simulink model "Verification_Tank1_Primitives"  (R2012b)
settings: Solver=FixedStepDiscrete  StartTime=0.0  StopTime=10.0  FixedStep=0.1  RelTol=1e-3
libraries: sldvlib x11
settings Model: Creator=Kerianne  LastModifiedBy=Kerianne
settings DataIOCC: SaveFormat=Structure
settings OptimizationCC: InlineParams=on

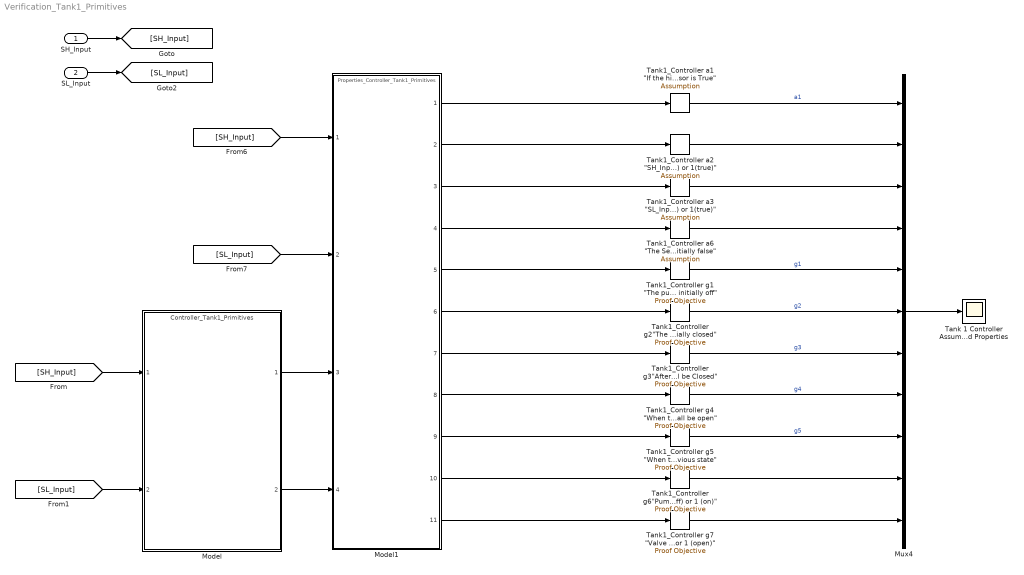
== system Verification_Tank1_Primitives ==
  SH_Input : Inport  OutDataTypeStr=double  SampleTime=0.1
  SL_Input : Inport  Port=2  OutDataTypeStr=double
  Model : ModelReference  ModelNameDialog=Controller_Tank1_Primitives  SimulationMode=Normal  ModelReferenceVersion=1.34  CopyOfModelName=Controller_Tank1_Primitives  DefaultDataLogging=on
  Model1 : ModelReference  ModelNameDialog=Properties_Controller_Tank1_Primitives  SimulationMode=Normal  ModelReferenceVersion=1.40  CopyOfModelName=Properties_Controller_Tank1_Primitives  DefaultDataLogging=on
  Mux4 : Mux  Inputs=11
  Tank 1 Controller Assumptions and Properties : Scope
      settings: ShowLegends=on  YMin=-1  YMax=2
  "Tank1_Controller a1 \"If the high sensor is true, then the low sensor is True\"" : sldvlib/Objectives and Constraints/Assumption  enabled=on  customAVTBlockType=Assumption  intervals=true  initial=off  dispValues=on  outEnabled=on
      settings: AttributesFormatString=%<intervals>
  "Tank1_Controller a2 \"SH_Input is 0 (false) or 1(true)\"" : sldvlib/Objectives and Constraints/Assumption  enabled=on  customAVTBlockType=Assumption  intervals=true  initial=off  dispValues=on  outEnabled=on
      settings: AttributesFormatString=%<intervals>
  "Tank1_Controller a3 \"SL_Input is 0 (false) or 1(true)\"" : sldvlib/Objectives and Constraints/Assumption  enabled=on  customAVTBlockType=Assumption  intervals=true  initial=off  dispValues=on  outEnabled=on
      settings: AttributesFormatString=%<intervals>
  "Tank1_Controller a6 \"The Sensors are initially false\"" : sldvlib/Objectives and Constraints/Assumption  enabled=on  customAVTBlockType=Assumption  intervals=true  initial=off  dispValues=on  outEnabled=on
      settings: AttributesFormatString=%<intervals>
  "Tank1_Controller g1 \"The pump is initially off\"" : sldvlib/Objectives and Constraints/Proof Objective  enabled=on  customAVTBlockType=Proof Objective  intervals=true  dispValues=on  outEnabled=on  enableStopSim=off
      settings: AttributesFormatString=%<intervals>
  "Tank1_Controller g2\"The valve is initially closed\"" : sldvlib/Objectives and Constraints/Proof Objective  enabled=on  customAVTBlockType=Proof Objective  intervals=true  dispValues=on  outEnabled=on  enableStopSim=off
      settings: AttributesFormatString=%<intervals>
  "Tank1_Controller g3\"After the initial time step, When SL_Input is False, the Pump shall be on and Valve shall be Closed\" " : sldvlib/Objectives and Constraints/Proof Objective  enabled=on  customAVTBlockType=Proof Objective  intervals=true  dispValues=on  outEnabled=on  enableStopSim=off
      settings: AttributesFormatString=%<intervals>
  "Tank1_Controller g4 \"When the SH_Input is true, the Pump shall be off and Valve shall be open\"" : sldvlib/Objectives and Constraints/Proof Objective  Description="\"The pump is initially off\""  enabled=on  customAVTBlockType=Proof Objective  intervals=true  dispValues=on  outEnabled=on  enableStopSim=off
      settings: AttributesFormatString=%<intervals>
  "Tank1_Controller g5 \"When the SL_Input is True and the SH_Input is False, the Pump and Valve shall stay in their previous state\"" : sldvlib/Objectives and Constraints/Proof Objective  Tag=g4  enabled=on  customAVTBlockType=Proof Objective  intervals=true  dispValues=on  outEnabled=on  enableStopSim=off
      settings: AttributesFormatString=%<intervals>
  "Tank1_Controller g6\"Pump State is 0 (off) or 1 (on)\"" : sldvlib/Objectives and Constraints/Proof Objective  Tag=g4  enabled=on  customAVTBlockType=Proof Objective  intervals=true  dispValues=on  outEnabled=on  enableStopSim=off
      settings: AttributesFormatString=%<intervals>
  "Tank1_Controller g7 \"Valve State is 0 (closed) or 1 (open)\"" : sldvlib/Objectives and Constraints/Proof Objective  Tag=g4  enabled=on  customAVTBlockType=Proof Objective  intervals=true  dispValues=on  outEnabled=on  enableStopSim=off
      settings: AttributesFormatString=%<intervals>
  wires:
  "Tank1_Controller a1 \"If the high sensor is true, then the low sensor is True\""/1 -> Mux4/1  "a1"
  "Tank1_Controller g4 \"When the SH_Input is true, the Pump shall be off and Valve shall be open\""/1 -> Mux4/8  "g4"
  "Tank1_Controller g1 \"The pump is initially off\""/1 -> Mux4/5  "g1"
  Model1/7 -> "Tank1_Controller g3\"After the initial time step, When SL_Input is False, the Pump shall be on and Valve shall be Closed\" "/1
  Model1/6 -> "Tank1_Controller g2\"The valve is initially closed\""/1
  Model1/5 -> "Tank1_Controller g1 \"The pump is initially off\""/1
  "Tank1_Controller g5 \"When the SL_Input is True and the SH_Input is False, the Pump and Valve shall stay in their previous state\""/1 -> Mux4/9  "g5"
  Model1/1 -> "Tank1_Controller a1 \"If the high sensor is true, then the low sensor is True\""/1
  "Tank1_Controller g2\"The valve is initially closed\""/1 -> Mux4/6  "g2"
  Mux4/1 -> Tank 1 Controller Assumptions and Properties/1
  Model1/8 -> "Tank1_Controller g4 \"When the SH_Input is true, the Pump shall be off and Valve shall be open\""/1
  Model1/10 -> "Tank1_Controller g6\"Pump State is 0 (off) or 1 (on)\""/1
  "Tank1_Controller g3\"After the initial time step, When SL_Input is False, the Pump shall be on and Valve shall be Closed\" "/1 -> Mux4/7  "g3"
  Model1/2 -> "Tank1_Controller a2 \"SH_Input is 0 (false) or 1(true)\""/1
  "Tank1_Controller a2 \"SH_Input is 0 (false) or 1(true)\""/1 -> Mux4/2
  "Tank1_Controller a3 \"SL_Input is 0 (false) or 1(true)\""/1 -> Mux4/3
  Model1/3 -> "Tank1_Controller a3 \"SL_Input is 0 (false) or 1(true)\""/1
  Model1/9 -> "Tank1_Controller g5 \"When the SL_Input is True and the SH_Input is False, the Pump and Valve shall stay in their previous state\""/1
  "Tank1_Controller g7 \"Valve State is 0 (closed) or 1 (open)\""/1 -> Mux4/11
  Model1/11 -> "Tank1_Controller g7 \"Valve State is 0 (closed) or 1 (open)\""/1
  "Tank1_Controller g6\"Pump State is 0 (off) or 1 (on)\""/1 -> Mux4/10
  Model/2 -> Model1/4
  Model/1 -> Model1/3
  SL_Input/1 -> [SL_Input]
  SH_Input/1 -> [SH_Input]
  [SH_Input] -> Model/1
  [SL_Input] -> Model/2
  [SH_Input] -> Model1/1
  [SL_Input] -> Model1/2
  Model1/4 -> "Tank1_Controller a6 \"The Sensors are initially false\""/1
  "Tank1_Controller a6 \"The Sensors are initially false\""/1 -> Mux4/4
